simulink model "temp"  (Simulink 7.7)
settings: Solver=ode45  StartTime=0.0  StopTime=10.0  RelTol=1e-3
undefined symbols (not defined in the file): DiscIntNeverNeededParam, g, I, lowSpd, M, R, T_veh, w0, w_max
settings Model: Creator=lfeng  LastModifiedBy=lfeng

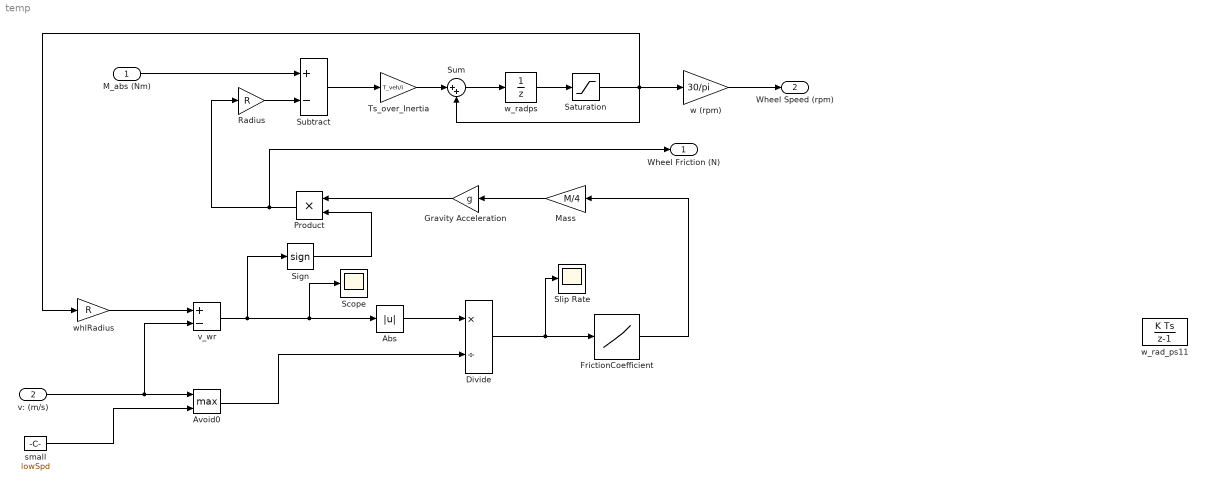
== system temp ==
  M_abs (Nm) : Inport
  v: (m/s) : Inport  Port=2
  Abs : Abs
  Avoid0 : MinMax  Function=max  Inputs=2
  Divide : Product  Inputs=*/
  FrictionCoefficient : Lookup  InputValues=[0 0.2 0.3 1]  Table=[0 0.3 0.2 0.2]  LookUpMeth=Interpolation-Use End Values  OutMin=0  OutMax=0.5
  Gravity Acceleration : Gain  Gain=g
  Mass : Gain  Gain=M/4
  Product : Product  RndMeth=Zero
  Radius : Gain  Gain=R
  Saturation : Saturate  UpperLimit=w_max  LowerLimit=0
  Scope : Scope
  Sign : Signum
  Slip Rate : Scope
  Subtract : Sum  Inputs=+-
  Sum : Sum  Inputs=|++
  Ts_over_Inertia : Gain  Gain=T_veh/I
  small : Constant  Value=lowSpd  OutMin=0.01  OutMax=1
  v_wr : Sum  Inputs=+-
  w (rpm) : Gain  Gain=30/pi  OutMin=0  OutMax=w_max*30/pi
  w_rad_ps11 : DiscreteIntegrator  InitialCondition=w0  SampleTime=-1  OutMin=0  OutMax=w_max  LimitOutput=on  UpperSaturationLimit=w_max  LowerSaturationLimit=0  ICPrevOutput=DiscIntNeverNeededParam  ICPrevScaledInput=DiscIntNeverNeededParam
  w_radps : UnitDelay  X0=w0  SampleTime=-1
  whlRadius : Gain  Gain=R  OutMin=0  OutMax=w_max/2
  Wheel Friction (N) : Outport
  Wheel Speed (rpm) : Outport  Port=2
  wires:
  M_abs (Nm)/1 -> Subtract/1
  v: (m/s)/1 -> Avoid0/1, v_wr/2
  w (rpm)/1 -> Wheel Speed (rpm)/1
  w_radps/1 -> Saturation/1
  Ts_over_Inertia/1 -> Sum/1
  Subtract/1 -> Ts_over_Inertia/1
  Radius/1 -> Subtract/2
  Mass/1 -> Gravity Acceleration/1
  Sign/1 -> Product/2
  Avoid0/1 -> Divide/2
  Gravity Acceleration/1 -> Product/1
  Product/1 -> Radius/1, Wheel Friction (N)/1
  v_wr/1 -> Sign/1, Abs/1, Scope/1
  Abs/1 -> Divide/1
  small/1 -> Avoid0/2
  whlRadius/1 -> v_wr/1
  Divide/1 -> FrictionCoefficient/1, Slip Rate/1
  FrictionCoefficient/1 -> Mass/1
  Sum/1 -> w_radps/1
  Saturation/1 -> w (rpm)/1, whlRadius/1, Sum/2
